simulink model "system_model"  (R2022b)
settings: Solver=VariableStepAuto  StartTime=0.0  StopTime=5  RelTol=1e-3
settings Model: Creator=SULTAN  LastModifiedBy=SULTAN

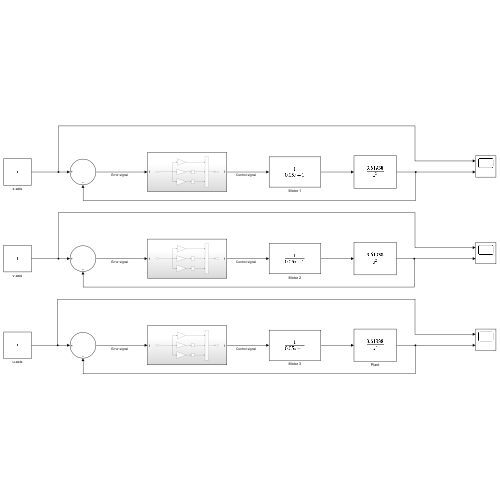
[thumbnail: Simulink's stored preview of the top-level diagram]
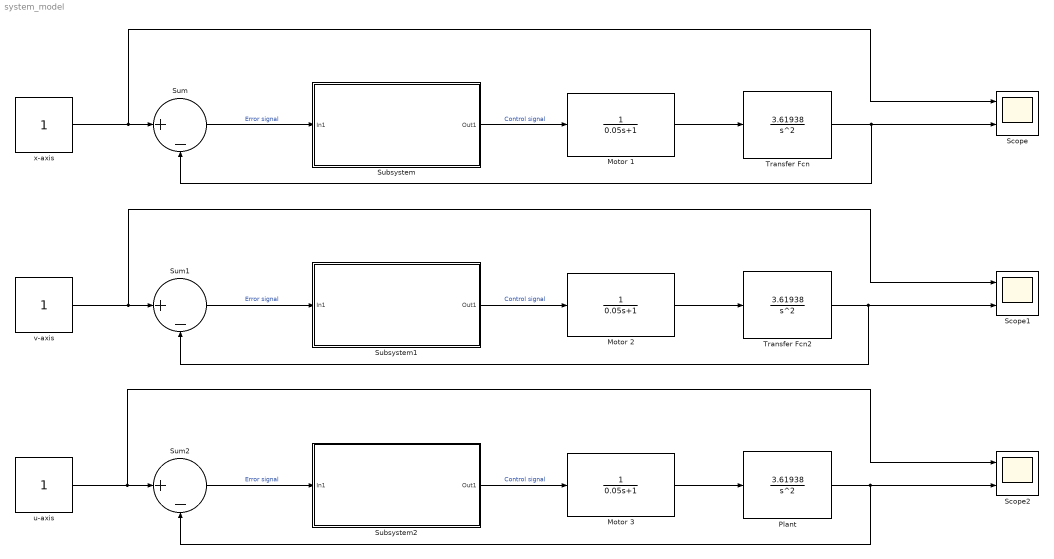
== system system_model ==
  Motor 1 : TransferFcn  Denominator=[0.05 1]
  Motor 2 : TransferFcn  Denominator=[0.05 1]
  Motor 3 : TransferFcn  Denominator=[0.05 1]
  Plant : TransferFcn  Numerator=[3.61938]  Denominator=[1 0 0]
  Scope : Scope  NumInputPorts=2
  Scope1 : Scope  NumInputPorts=2
  Scope2 : Scope  NumInputPorts=2
  Subsystem : Subsystem
  Subsystem1 : Subsystem
  Subsystem2 : Subsystem
  Sum : Sum  Inputs=|+-
  Sum1 : Sum  Inputs=|+-
  Sum2 : Sum  Inputs=|+-
  Transfer Fcn : TransferFcn  Numerator=[3.61938]  Denominator=[1 0 0]
  Transfer Fcn2 : TransferFcn  Numerator=[3.61938]  Denominator=[1 0 0]
  u-axis : Constant
  v-axis : Constant
  x-axis : Constant
  wires:
  Transfer Fcn/1 -> Scope/2, Sum/2
  Motor 1/1 -> Transfer Fcn/1
  x-axis/1 -> Scope/1, Sum/1
  Sum/1 -> Subsystem/1(In1)  "Error signal"
  Subsystem/1(Out1) -> Motor 1/1  "Control signal"
  Subsystem1/1(Out1) -> Motor 2/1  "Control signal"
  Sum1/1 -> Subsystem1/1(In1)  "Error signal"
  v-axis/1 -> Scope1/1, Sum1/1
  Transfer Fcn2/1 -> Scope1/2, Sum1/2
  Motor 2/1 -> Transfer Fcn2/1
  Subsystem2/1(Out1) -> Motor 3/1  "Control signal"
  Sum2/1 -> Subsystem2/1(In1)  "Error signal"
  u-axis/1 -> Scope2/1, Sum2/1
  Plant/1 -> Scope2/2, Sum2/2
  Motor 3/1 -> Plant/1

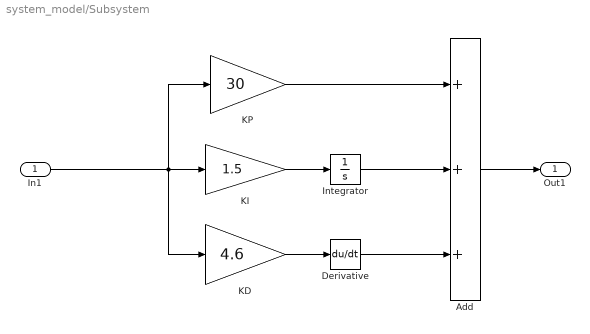
== system system_model/Subsystem ==
  In1 : Inport
  Add : Sum  Inputs=+++
  Derivative : Derivative
  Integrator : Integrator
  KD : Gain  Gain=4.6
  KI : Gain  Gain=1.5
  KP : Gain  Gain=30
  Out1 : Outport
  wires:
  Add/1 -> Out1/1
  In1/1 -> KP/1, KD/1, KI/1
  KD/1 -> Derivative/1
  Derivative/1 -> Add/3
  KI/1 -> Integrator/1
  KP/1 -> Add/1
  Integrator/1 -> Add/2

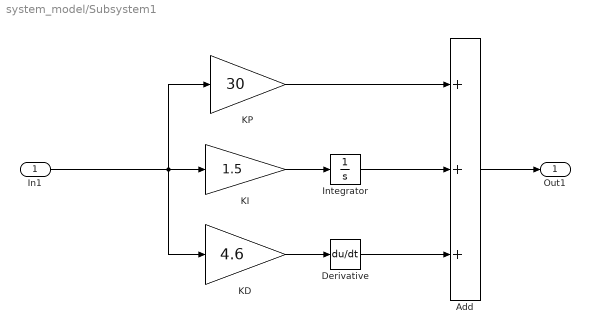
== system system_model/Subsystem1 ==
  In1 : Inport
  Add : Sum  Inputs=+++
  Derivative : Derivative
  Integrator : Integrator
  KD : Gain  Gain=4.6
  KI : Gain  Gain=1.5
  KP : Gain  Gain=30
  Out1 : Outport
  wires:
  Add/1 -> Out1/1
  In1/1 -> KP/1, KD/1, KI/1
  KD/1 -> Derivative/1
  Derivative/1 -> Add/3
  KI/1 -> Integrator/1
  KP/1 -> Add/1
  Integrator/1 -> Add/2

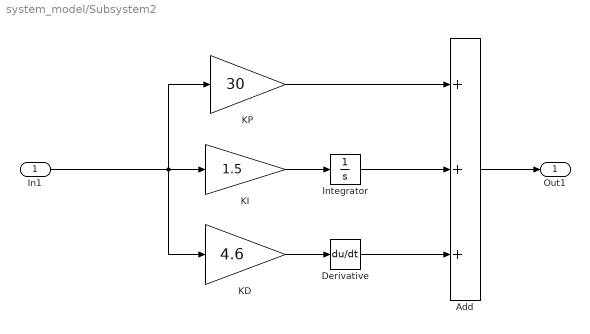
== system system_model/Subsystem2 ==
  In1 : Inport
  Add : Sum  Inputs=+++
  Derivative : Derivative
  Integrator : Integrator
  KD : Gain  Gain=4.6
  KI : Gain  Gain=1.5
  KP : Gain  Gain=30
  Out1 : Outport
  wires:
  Add/1 -> Out1/1
  In1/1 -> KP/1, KD/1, KI/1
  KD/1 -> Derivative/1
  Derivative/1 -> Add/3
  KI/1 -> Integrator/1
  KP/1 -> Add/1
  Integrator/1 -> Add/2
